simulink model "Lab_1"  (R2022b)
settings: Solver=VariableStepAuto  StartTime=0.0  StopTime=10.0  RelTol=1e-3
settings Model: Creator=MOHAMED  LastModifiedBy=MOHAMED

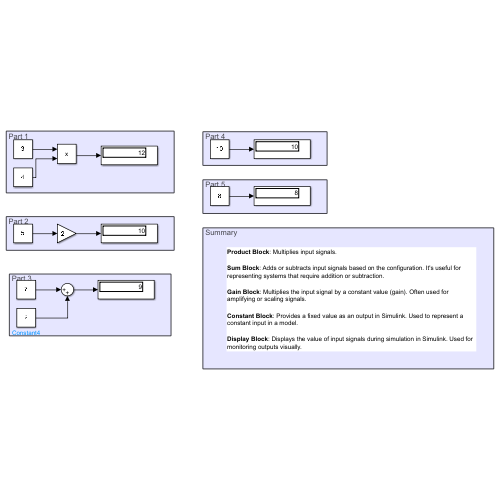
[thumbnail: Simulink's stored preview of the top-level diagram]
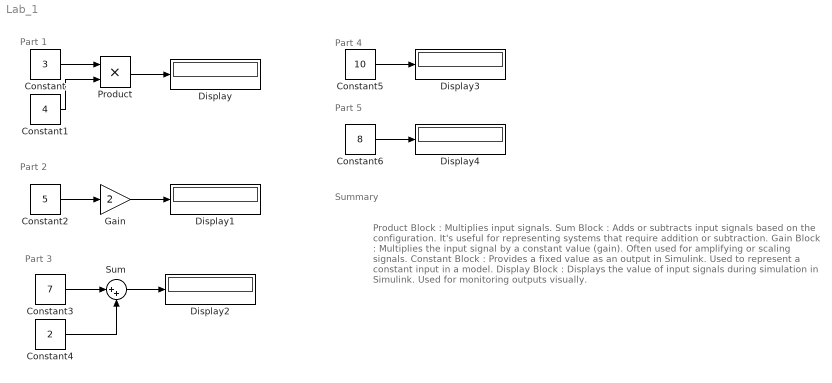
== system Lab_1 ==
  note: Summary
  note: Product Block : Multiplies input signals.
      |
      | Sum Block : Adds or subtracts input signals based on the configuration. It's useful for representing systems that require addition or subtraction.
      |
      | Gain Block : Multiplies the input signal by a constant value (gain). Often used for amplifying or scaling signals.
      |
      | Constant Block : Provides a fixed value as an output in Simulink. Used to represent a constant input in a model.
      |
      | Display Block : Displays the value of input signals during simulation in Simulink. Used for monitoring outputs visually.
  note: Part 5
  note: Part 4
  note: Part 3
  note: Part 2
  note: Part 1
  Constant : Constant  Value=3
  Constant1 : Constant  Value=4
  Constant2 : Constant  Value=5
  Constant3 : Constant  Value=7
  Constant4 : Constant  Value=2
  Constant5 : Constant  Value=10
  Constant6 : Constant  Value=8
  Display{,1..4} (5 alike) : Display
  Gain : Gain  Gain=2
  Product : Product
  Sum : Sum  Inputs=|++
  wires:
  Constant6/1 -> Display4/1
  Constant1/1 -> Product/2
  Constant/1 -> Product/1
  Sum/1 -> Display2/1
  Constant2/1 -> Gain/1
  Product/1 -> Display/1
  Constant3/1 -> Sum/1
  Constant5/1 -> Display3/1
  Constant4/1 -> Sum/2
  Gain/1 -> Display1/1
